simulink model "simulazione_definitiva"  (R2024b)
settings: Solver=VariableStepAuto  StartTime=0.0  StopTime=15  RelTol=1e-3
values from neighbouring files (symbols this model uses):
  A4 = horzcat([0;0;0;0], A4)    [forwarding.m]    (also in stabilita_AS.m)
  BB = [0; B_sub]    [forwarding.m]    (also in stabilita_AS.m = [0; B])
  KK = [0 K_sub]    [forwarding.m]    (also in stabilita_AS.m = [0 K])
  L_oss = (1/epsilon) * L0    [forwarding.m]    (also in stabilita_AS.m)
settings Model: Creator=costa  LastModifiedBy=costa

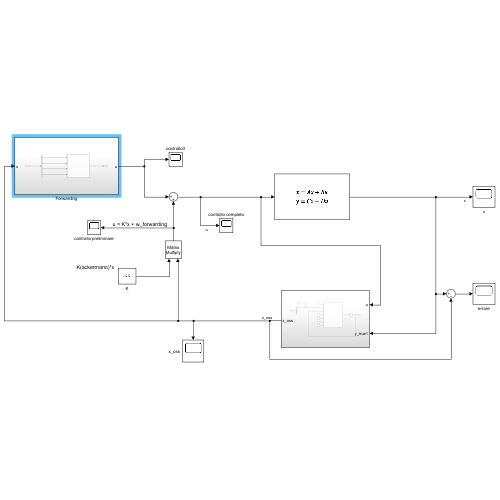
[thumbnail: Simulink's stored preview of the top-level diagram]
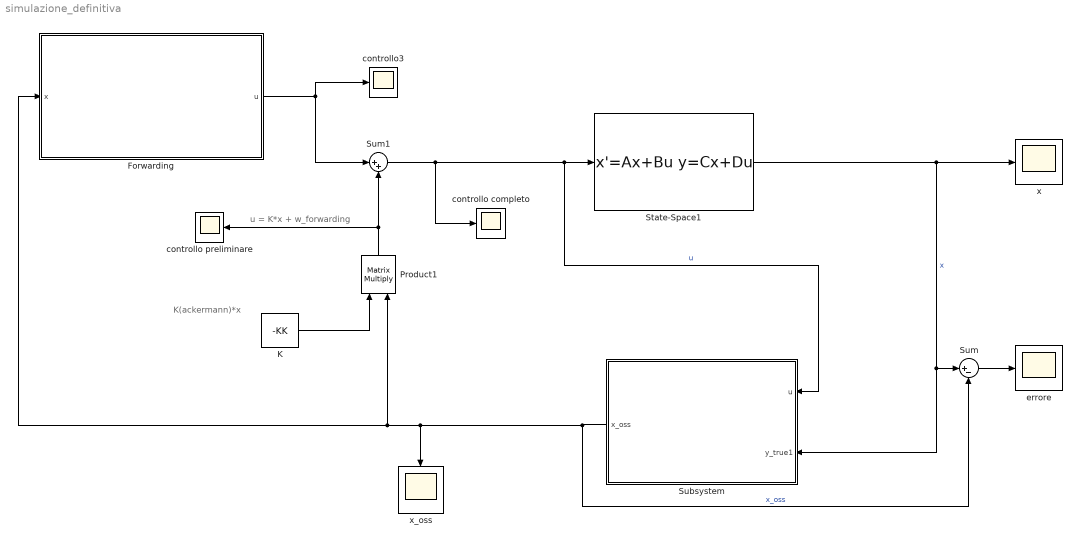
== system simulazione_definitiva ==
  note: K(ackermann)*x
  note: u = K*x + w_forwarding
  Forwarding : Subsystem
  K : Constant  Value=-KK  VectorParams1D=off
  Product1 : Product  Multiplication=Matrix(*)
  State-Space1 : StateSpace  A=A4  B=BB  C=eye(4)  D=[0; 0; 0; 0]  InitialCondition=[1, 2 , 3, 0]
  Subsystem : Subsystem
  Sum : Sum  Inputs=|+-
  Sum1 : Sum  Inputs=|++
  controllo completo : Scope
  controllo preliminare : Scope
  controllo3 : Scope
  errore : Scope
  x : Scope
  x_oss : Scope
  wires:
  Sum1/1 -> controllo completo/1, Subsystem/1(u), State-Space1/1  "u"
  K/1 -> Product1/1
  Product1/1 -> controllo preliminare/1, Sum1/2
  State-Space1/1 -> x/1, Subsystem/2(y_true1), Sum/1  "x"
  Forwarding/1(u) -> controllo3/1, Sum1/1
  Subsystem/1(x_oss) -> Sum/2, Product1/2, Forwarding/1(x), x_oss/1  "x_oss"
  Sum/1 -> errore/1

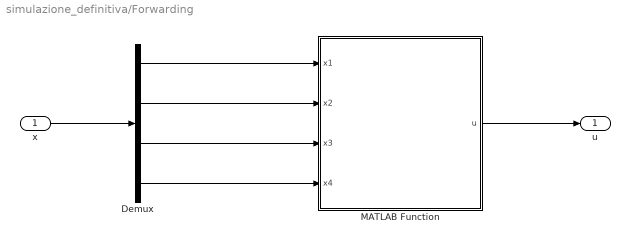
== system simulazione_definitiva/Forwarding ==
  x : Inport
  Demux : Demux
  MATLAB Function : MATLAB Function  TreatAsAtomicUnit=on
  u : Outport
  wires:
  MATLAB Function/1(u) -> u/1
  x/1 -> Demux/1
  Demux/1 -> MATLAB Function/1(x1)
  Demux/2 -> MATLAB Function/2(x2)
  Demux/3 -> MATLAB Function/3(x3)
  Demux/4 -> MATLAB Function/4(x4)

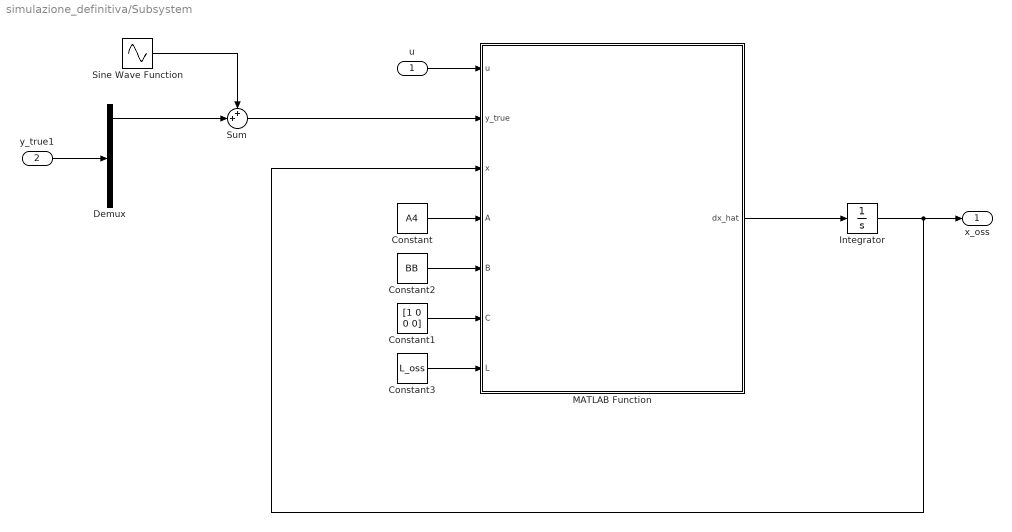
== system simulazione_definitiva/Subsystem ==
  u : Inport
  y_true1 : Inport  Port=2
  Constant : Constant  Value=A4  VectorParams1D=off
  Constant1 : Constant  Value=[1 0 0 0]  VectorParams1D=off
  Constant2 : Constant  Value=BB  VectorParams1D=off
  Constant3 : Constant  Value=L_oss  VectorParams1D=off
  Demux : Demux
  Integrator : Integrator  InitialCondition=[0 0 0 0]
  MATLAB Function : MATLAB Function  TreatAsAtomicUnit=on
  Sine Wave Function : Sin  TimeSource=Use external signal  Amplitude=0.1  Frequency=2*pi*50  SampleTime=0
  Sum : Sum  Inputs=++|
  x_oss : Outport
  wires:
  u/1 -> MATLAB Function/1(u)
  MATLAB Function/1(dx_hat) -> Integrator/1
  Constant1/1 -> MATLAB Function/6(C)
  Constant2/1 -> MATLAB Function/5(B)
  Constant/1 -> MATLAB Function/4(A)
  Constant3/1 -> MATLAB Function/7(L)
  Sum/1 -> MATLAB Function/2(y_true)
  Sine Wave Function/1 -> Sum/1
  Integrator/1 -> MATLAB Function/3(x), x_oss/1
  y_true1/1 -> Demux/1
  Demux/1 -> Sum/2

== matlab function simulazione_definitiva/Forwarding/MATLAB Function ==
  data: x1 input; u output; x2 input; x3 input; x4 input
function u = fcn(x1, x2, x3, x4)

    x1_des = 1;
    u = (2725*x1)/6 + (29975*x2)/36 - (59405*x3)/6 - (59405*x4)/36 - (2725*x1_des)/6 - 125*0.01*((11931*x3)/250 - (109*x2)/30 + (12181*x4)/1500);

end

== matlab function simulazione_definitiva/Subsystem/MATLAB Function ==
  data: u input; dx_hat output; y_true input; x input; A input; B input; C input; L input
function dx_hat = fcn(u, y_true, x, A, B, C, L)
    disp(size(y_true))
    dx_hat = A*x + B*u + L*(y_true-C*x);
end
